simulink model "ParmTblWValidation"  (R2018b)
settings: Solver=FixedStepDiscrete  StartTime=0.0  StopTime=10  FixedStep=.01  RelTol=1e-3
PostLoadFcn:
  | load test_data.mat;
undefined symbols (not defined in the file or in its folder): parmTbl, parmTblWVal
settings Model: TunableVars=B,K  TunableVarsStorageClass=Auto,Auto  TunableVarsTypeQualifier=,  Creator=mmcbroom  LastModifiedBy=slentine
settings DataIOCC: LimitDataPoints=on  SaveFormat=StructureWithTime  SignalLoggingSaveFormat=ModelDataLogs  SaveOutput=off  SignalLogging=off  SaveTime=off
settings OptimizationCC: DefaultParameterBehavior=Inlined  EnhancedBackFolding=on  PassReuseOutputArgsAs=Individual arguments  ExpressionDepthLimit=2147483647  InitFltsAndDblsToZero=on  OptimizeBlockOrder=speed  DifferentSizesBufferReuse=on  OptimizationCustomize=off
settings DebuggingCC: MergeDetectMultiDrivingBlocksExec=none  SolverPrmCheckMsg=warning  ParameterTunabilityLossMsg=error  FcnCallInpInsideContextMsg=warning  BusObjectLabelMismatch=error  StateNameClashWarn=warning  StrictBusMsg=WarnOnBusTreatedAsVector  SFUnexpectedBacktrackingDiag=warning  SFNoUnconditionalDefaultTransitionDiag=warning  SFExecutionAtInitializationDiag=none
settings HardwareCC: ProdBitPerPointer=32  ProdBitPerSizeT=32  ProdBitPerPtrDiffT=32  ProdLargestAtomicFloat=None  ProdIntDivRoundTo=Undefined  ProdEndianess=Unspecified  ProdWordSize=32  ProdHWDeviceType=32-bit Generic
settings ModelReferenceCC: PropagateSignalLabelsOutOfModel=off
settings SFSimCC: SimUseLocalCustomCode=off  MATLABDynamicMemAlloc=off
settings RTWCC: SystemTargetFile=cfs_ert.tlc  TemplateMakefile=ert_default_tmf  Description=NASA CFS Target File  GenerateReport=on  RTWUseLocalCustomCode=off  IncludeHyperlinkInReport=on  LaunchReport=on  PortableWordSizes=on  GenerateTraceInfo=on  GenerateTraceReport=on  GenerateTraceReportSl=on  GenerateTraceReportSf=on  GenerateTraceReportEml=on
settings CodeAppCC: ForceParamTrailComments=on  IgnoreCustomStorageClasses=off  OperatorAnnotations=on  SimulinkDataObjDesc=on  SFDataObjDesc=on  CustomSymbolStrType=$N$R$M  InsertBlockDesc=on  InternalIdentifier=Classic  ReqsInCode=on
settings STFCustomTargetCC: MultiwordLength=256  GenerateSampleERTMain=on  CombineOutputUpdateFcns=on  ERTCustomFileBanners=on  SupportContinuousTime=off  SupportNonInlinedSFcns=off  RemoveResetFunc=on  MATLABClassNameForMDSCustomization=Simulink.SoftwareTarget.ERTCustomization  UseToolchainInfoCompliant=on  SystemTargetFile=cfs_ert.tlc
settings ERTTargetCC: GenerateSampleERTMain=on  ParMdlRefBuildCompliant=off  CompOptLevelCompliant=off  ConcurrentExecutionCompliant=off  ModelStepFunctionPrototypeControlCompliant=off  CPPClassGenCompliant=off  InlinedParameterPlacement=NonHierarchical  ERTCustomFileTemplate=cfs_interface.tlc
settings ConfigComp: CovMetricSettings=dw  CovHtmlReporting=on  CovSaveCumulativeToWorkspaceVar=on  CovSaveSingleToWorkspaceVar=on  CovExternalEMLEnable=off  CovSFcnEnable=off

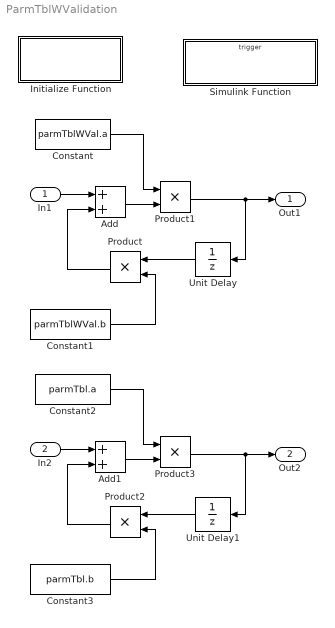
== system ParmTblWValidation ==
  In1 : Inport  BusOutputAsStruct=on
  In2 : Inport  Port=2  BusOutputAsStruct=on
  Add : Sum
  Add1 : Sum
  Constant : Constant  Value=parmTblWVal.a
  Constant1 : Constant  Value=parmTblWVal.b
  Constant2 : Constant  Value=parmTbl.a
  Constant3 : Constant  Value=parmTbl.b
  Initialize Function : Subsystem  TreatAsAtomicUnit=on
  Product{,1..3} (4 alike) : Product
  Simulink Function : Subsystem  TreatAsAtomicUnit=on
  Unit Delay : UnitDelay  SampleTime=-1
  Unit Delay1 : UnitDelay  SampleTime=-1
  Out1 : Outport
  Out2 : Outport  Port=2
  wires:
  In1/1 -> Add/1
  Product1/1 -> Unit Delay/1, Out1/1
  Add/1 -> Product1/2
  Product/1 -> Add/2
  Unit Delay/1 -> Product/1
  Constant1/1 -> Product/2
  Constant/1 -> Product1/1
  Constant2/1 -> Product3/1
  Constant3/1 -> Product2/2
  Unit Delay1/1 -> Product2/1
  Product2/1 -> Add1/2
  Add1/1 -> Product3/2
  Product3/1 -> Out2/1, Unit Delay1/1
  In2/1 -> Add1/1

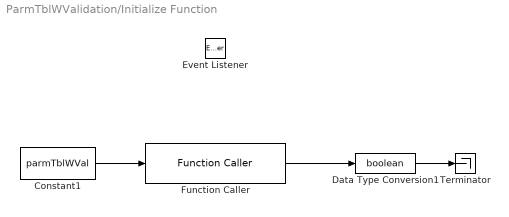
== system ParmTblWValidation/Initialize Function ==
  Constant1 : Constant  Value=parmTblWVal  OutDataTypeStr=Bus: parmTbl_b
  Data Type Conversion1 : DataTypeConversion  OutDataTypeStr=boolean
  Event Listener : EventListener  DisableCoverage=on  EventName=reset
  Function Caller : FunctionCaller  FunctionPrototype=retVal = tblValFcn_f(tbl)
  Terminator : Terminator
  wires:
  Constant1/1 -> Function Caller/1
  Function Caller/1 -> Data Type Conversion1/1
  Data Type Conversion1/1 -> Terminator/1

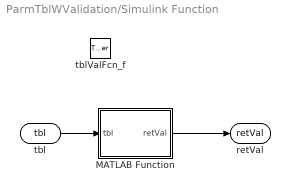
== system ParmTblWValidation/Simulink Function ==
  tblValFcn_f : TriggerPort  TriggerType=function-call  IsSimulinkFunction=on  FunctionName=tblValFcn_f  VariantControl=(inherit)
  MATLAB Function : MATLAB Function  TreatAsAtomicUnit=on
  tbl : ArgIn  DisableCoverage=on  OutDataTypeStr=Bus: parmTbl_b  ArgumentName=tbl
  retVal : ArgOut  DisableCoverage=on  OutDataTypeStr=int32  ArgumentName=retVal
  wires:
  tbl/1 -> MATLAB Function/1(tbl)
  MATLAB Function/1(retVal) -> retVal/1

== matlab function ParmTblWValidation/Simulink Function/MATLAB Function ==
  data: tbl input; retVal output
function retVal = fcn(tbl)

    retVal = tblValFcn(tbl);
    
end
